simulink model "rotor_model_c"  (R2016a)
settings: Solver=VariableStepAuto  StartTime=0.0  StopTime=10.0  RelTol=1e-3
undefined symbols (not defined in the file): Am, Ap, B, x0
settings Model: Creator=mgreiff  LastModifiedBy=mgreiff
settings DataIOCC: LimitDataPoints=on
settings DebuggingCC: AllowSymbolicDim=off
settings ModelReferenceCC: PropagateSignalLabelsOutOfModel=off
settings GRTTargetCC: GeneratePreprocessorConditionals=Use local settings

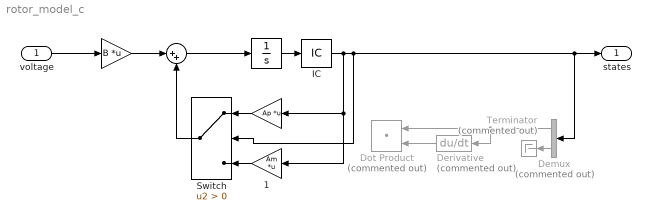
== system rotor_model_c ==
  voltage : Inport  PortDimensions=1
  " " : Sum  Inputs=|++
  "  " : Gain  Gain=B  Multiplication=Matrix(K*u)
  "   " : Integrator
  "    " : Gain  Gain=Ap  Multiplication=Matrix(K*u)
  "    1" : Gain  Gain=Am  Multiplication=Matrix(K*u)
  Demux : Demux  Commented=on  Outputs=2
  Derivative : Derivative  Commented=on
  Dot Product : DotProduct  Commented=on  InputSameDT=on  OutDataTypeStr=Inherit: Inherit via internal rule
  IC : InitialCondition  Value=x0
  Switch : Switch  Criteria=u2 > Threshold
  Terminator : Terminator  Commented=on
  states : Outport
  wires:
  voltage/1 -> "  "/1
  " "/1 -> "   "/1
  "  "/1 -> " "/1
  "   "/1 -> IC/1
  IC/1 -> "    1"/1, "    "/1, Switch/2, Demux/1, states/1
  "    "/1 -> Switch/1
  "    1"/1 -> Switch/3
  Demux/2 -> Terminator/1
  Switch/1 -> " "/2
  Demux/1 -> Derivative/1, Dot Product/1
  Derivative/1 -> Dot Product/2
